simulink model "ProgramCounter"  (R2025b)
settings: Solver=VariableStepAuto  StartTime=0.0  StopTime=10.0  RelTol=1e-3
libraries: dspsigops x1
settings Model: Creator=cyber  LastModifiedBy=cyber

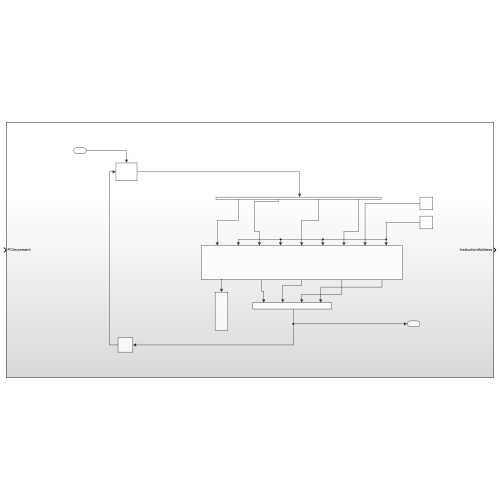
[thumbnail: Simulink's stored preview of the top-level diagram]
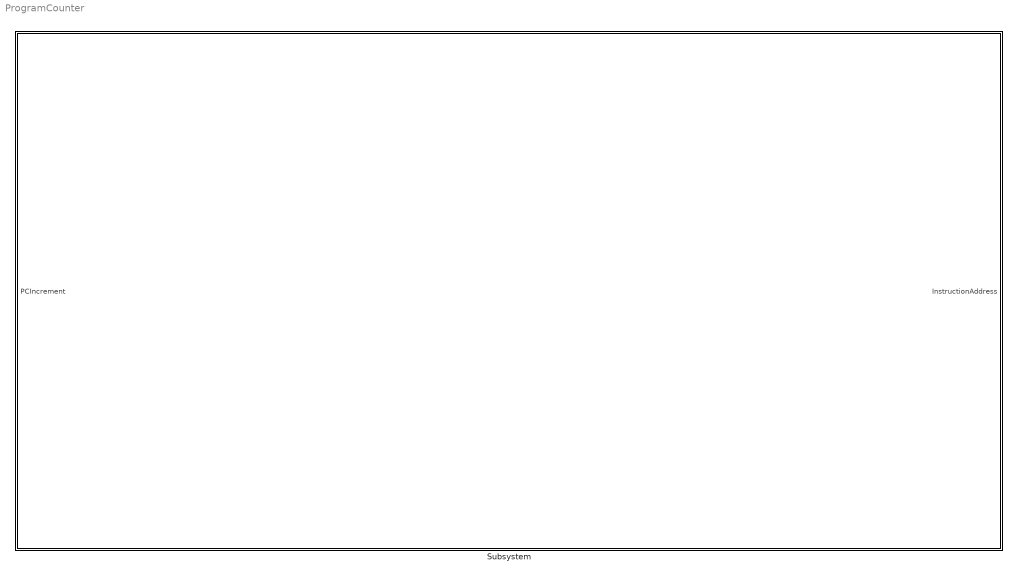
== system ProgramCounter ==
  Subsystem : Subsystem

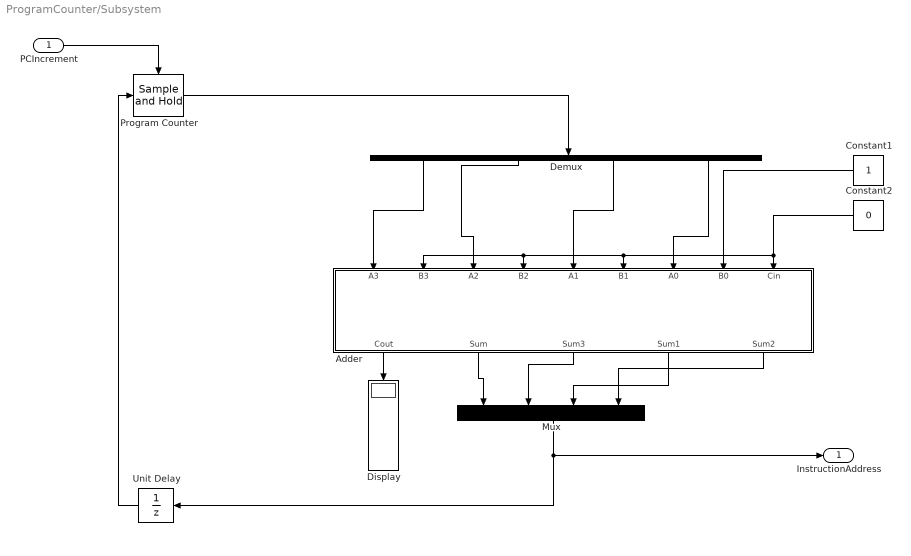
== system ProgramCounter/Subsystem ==
  PCIncrement : Inport
  Adder : Subsystem
  Constant1 : Constant
  Constant2 : Constant  Value=0
  Demux : Demux
  Display : Display
  Mux : Mux
  Program Counter : dspsigops/Sample and Hold  trig=Rising edge  initCond=0  latchinput=off
  Unit Delay : UnitDelay  SampleTime=-1  HasFrameUpgradeWarning=on
  InstructionAddress : Outport
  wires:
  Constant2/1 -> Adder/2(B3), Adder/4(B2), Adder/6(B1), Adder/9(Cin)
  Demux/2 -> Adder/3(A2)
  PCIncrement/1 -> Program Counter/Trigger
  Constant1/1 -> Adder/8(B0)
  Demux/3 -> Adder/5(A1)
  Program Counter/1 -> Demux/1
  Demux/4 -> Adder/7(A0)
  Demux/1 -> Adder/1(A3)
  Adder/2(Sum) -> Mux/1
  Adder/1(Cout) -> Display/1
  Unit Delay/1 -> Program Counter/1
  Mux/1 -> InstructionAddress/1, Unit Delay/1
  Adder/5(Sum2) -> Mux/4
  Adder/3(Sum3) -> Mux/2
  Adder/4(Sum1) -> Mux/3

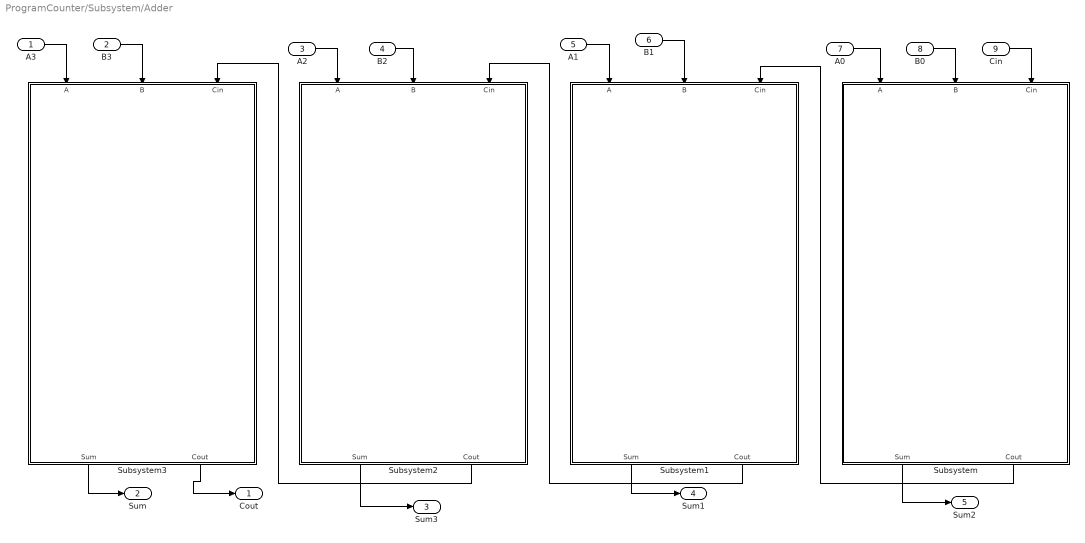
== system ProgramCounter/Subsystem/Adder ==
  A3 : Inport
  B3 : Inport  Port=2
  A2 : Inport  Port=3
  B2 : Inport  Port=4
  A1 : Inport  Port=5
  B1 : Inport  Port=6
  A0 : Inport  Port=7
  B0 : Inport  Port=8
  Cin : Inport  Port=9
  Subsystem : Subsystem
  Subsystem1 : Subsystem
  Subsystem2 : Subsystem
  Subsystem3 : Subsystem
  Cout : Outport
  Sum : Outport  Port=2
  Sum3 : Outport  Port=3
  Sum1 : Outport  Port=4
  Sum2 : Outport  Port=5
  wires:
  Subsystem2/2(Cout) -> Subsystem3/3(Cin)
  B3/1 -> Subsystem3/2(B)
  Subsystem/2(Cout) -> Subsystem1/3(Cin)
  A2/1 -> Subsystem2/1(A)
  A3/1 -> Subsystem3/1(A)
  A1/1 -> Subsystem1/1(A)
  Subsystem/1(Sum) -> Sum2/1
  Subsystem1/2(Cout) -> Subsystem2/3(Cin)
  B1/1 -> Subsystem1/2(B)
  B0/1 -> Subsystem/2(B)
  Subsystem3/1(Sum) -> Sum/1
  B2/1 -> Subsystem2/2(B)
  Subsystem1/1(Sum) -> Sum1/1
  Subsystem2/1(Sum) -> Sum3/1
  Cin/1 -> Subsystem/3(Cin)
  Subsystem3/2(Cout) -> Cout/1
  A0/1 -> Subsystem/1(A)

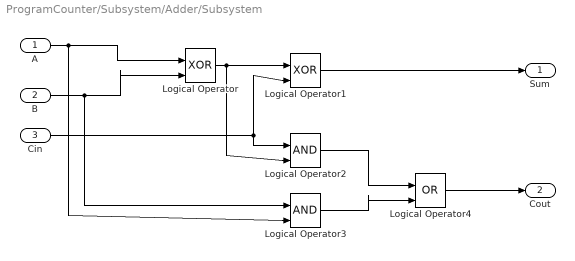
== system ProgramCounter/Subsystem/Adder/Subsystem ==
  A : Inport
  B : Inport  Port=2
  Cin : Inport  Port=3
  Logical Operator : Logic  Operator=XOR  IconShape=distinctive  AllPortsSameDT=off  OutDataTypeStr=boolean
  Logical Operator1 : Logic  Operator=XOR  IconShape=distinctive  AllPortsSameDT=off  OutDataTypeStr=boolean
  Logical Operator2 : Logic  IconShape=distinctive  AllPortsSameDT=off  OutDataTypeStr=boolean
  Logical Operator3 : Logic  IconShape=distinctive  AllPortsSameDT=off  OutDataTypeStr=boolean
  Logical Operator4 : Logic  Operator=OR  IconShape=distinctive  AllPortsSameDT=off  OutDataTypeStr=boolean
  Sum : Outport
  Cout : Outport  Port=2
  wires:
  B/1 -> Logical Operator3/1, Logical Operator/2
  Logical Operator1/1 -> Sum/1
  Logical Operator3/1 -> Logical Operator4/2
  Logical Operator/1 -> Logical Operator2/2, Logical Operator1/1
  Logical Operator4/1 -> Cout/1
  Cin/1 -> Logical Operator2/1, Logical Operator1/2
  Logical Operator2/1 -> Logical Operator4/1
  A/1 -> Logical Operator3/2, Logical Operator/1

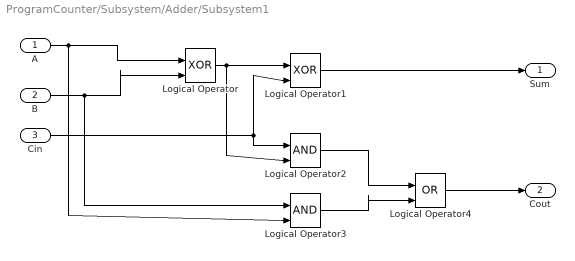
== system ProgramCounter/Subsystem/Adder/Subsystem1 ==
  A : Inport
  B : Inport  Port=2
  Cin : Inport  Port=3
  Logical Operator : Logic  Operator=XOR  IconShape=distinctive  AllPortsSameDT=off  OutDataTypeStr=boolean
  Logical Operator1 : Logic  Operator=XOR  IconShape=distinctive  AllPortsSameDT=off  OutDataTypeStr=boolean
  Logical Operator2 : Logic  IconShape=distinctive  AllPortsSameDT=off  OutDataTypeStr=boolean
  Logical Operator3 : Logic  IconShape=distinctive  AllPortsSameDT=off  OutDataTypeStr=boolean
  Logical Operator4 : Logic  Operator=OR  IconShape=distinctive  AllPortsSameDT=off  OutDataTypeStr=boolean
  Sum : Outport
  Cout : Outport  Port=2
  wires:
  B/1 -> Logical Operator3/1, Logical Operator/2
  Logical Operator1/1 -> Sum/1
  Logical Operator3/1 -> Logical Operator4/2
  Logical Operator/1 -> Logical Operator2/2, Logical Operator1/1
  Logical Operator4/1 -> Cout/1
  Cin/1 -> Logical Operator2/1, Logical Operator1/2
  Logical Operator2/1 -> Logical Operator4/1
  A/1 -> Logical Operator3/2, Logical Operator/1

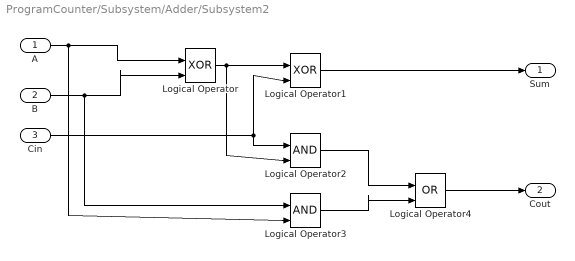
== system ProgramCounter/Subsystem/Adder/Subsystem2 ==
  A : Inport
  B : Inport  Port=2
  Cin : Inport  Port=3
  Logical Operator : Logic  Operator=XOR  IconShape=distinctive  AllPortsSameDT=off  OutDataTypeStr=boolean
  Logical Operator1 : Logic  Operator=XOR  IconShape=distinctive  AllPortsSameDT=off  OutDataTypeStr=boolean
  Logical Operator2 : Logic  IconShape=distinctive  AllPortsSameDT=off  OutDataTypeStr=boolean
  Logical Operator3 : Logic  IconShape=distinctive  AllPortsSameDT=off  OutDataTypeStr=boolean
  Logical Operator4 : Logic  Operator=OR  IconShape=distinctive  AllPortsSameDT=off  OutDataTypeStr=boolean
  Sum : Outport
  Cout : Outport  Port=2
  wires:
  B/1 -> Logical Operator3/1, Logical Operator/2
  Logical Operator1/1 -> Sum/1
  Logical Operator3/1 -> Logical Operator4/2
  Logical Operator/1 -> Logical Operator2/2, Logical Operator1/1
  Logical Operator4/1 -> Cout/1
  Cin/1 -> Logical Operator2/1, Logical Operator1/2
  Logical Operator2/1 -> Logical Operator4/1
  A/1 -> Logical Operator3/2, Logical Operator/1

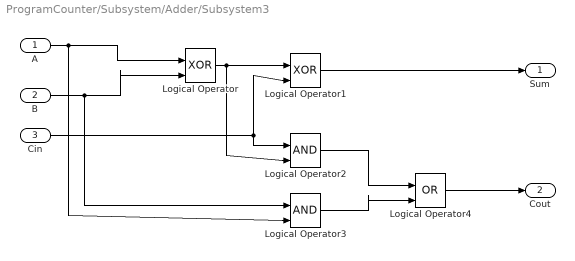
== system ProgramCounter/Subsystem/Adder/Subsystem3 ==
  A : Inport
  B : Inport  Port=2
  Cin : Inport  Port=3
  Logical Operator : Logic  Operator=XOR  IconShape=distinctive  AllPortsSameDT=off  OutDataTypeStr=boolean
  Logical Operator1 : Logic  Operator=XOR  IconShape=distinctive  AllPortsSameDT=off  OutDataTypeStr=boolean
  Logical Operator2 : Logic  IconShape=distinctive  AllPortsSameDT=off  OutDataTypeStr=boolean
  Logical Operator3 : Logic  IconShape=distinctive  AllPortsSameDT=off  OutDataTypeStr=boolean
  Logical Operator4 : Logic  Operator=OR  IconShape=distinctive  AllPortsSameDT=off  OutDataTypeStr=boolean
  Sum : Outport
  Cout : Outport  Port=2
  wires:
  B/1 -> Logical Operator3/1, Logical Operator/2
  Logical Operator1/1 -> Sum/1
  Logical Operator3/1 -> Logical Operator4/2
  Logical Operator/1 -> Logical Operator2/2, Logical Operator1/1
  Logical Operator4/1 -> Cout/1
  Cin/1 -> Logical Operator2/1, Logical Operator1/2
  Logical Operator2/1 -> Logical Operator4/1
  A/1 -> Logical Operator3/2, Logical Operator/1
